simulink model "KF"  (R2021b)
settings: Solver=VariableStepAuto  StartTime=0.0  StopTime=10.0  RelTol=1e-3
values from neighbouring files (symbols this model uses):
  AA = [0 1; g/L 0]    [simConstants.m]
  BB = [0; -1/L]    [simConstants.m]
  CC = [1 0]    [simConstants.m]
  K = W * CC' / V2    [simConstants.m]
libraries: simulink_extras x4
settings Model: Creator=logan  LastModifiedBy=logan

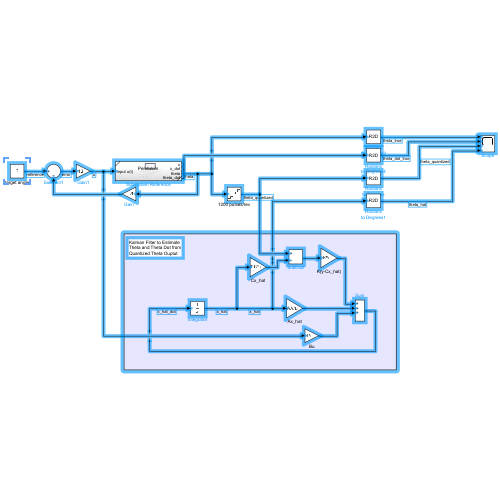
[thumbnail: Simulink's stored preview of the top-level diagram]
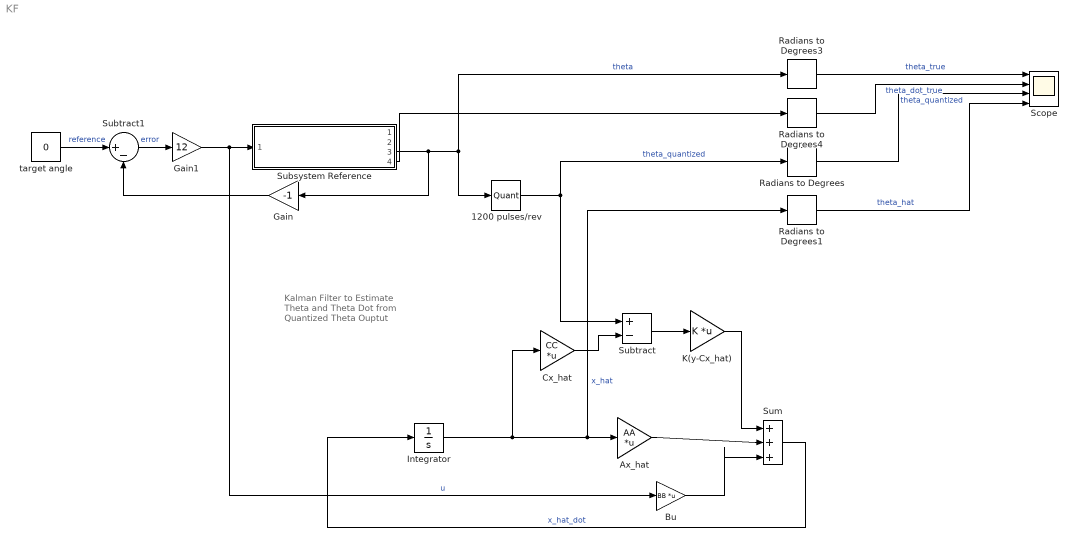
== system KF ==
  note: Kalman Filter to Estimate
      | Theta and Theta Dot from
      | Quantized Theta Ouptut
  1200 pulses/rev : Quantizer  QuantizationInterval=(2*pi)/1200
  Ax_hat : Gain  Gain=AA  Multiplication=Matrix(K*u)
  Bu : Gain  Gain=BB  Multiplication=Matrix(K*u)
  Cx_hat : Gain  Gain=CC  Multiplication=Matrix(K*u)
  Gain : Gain  Gain=-1
  Gain1 : Gain  Gain=12
  Integrator : Integrator
  K(y-Cx_hat) : Gain  Gain=K  Multiplication=Matrix(K*u)
  Radians to Degrees{,1,3..4} (4 alike) : simulink_extras/Transformations/Radians to Degrees
  Scope : Scope  NumInputPorts=4
  Subsystem Reference : Subsystem  ReferencedSubsystem=Pendulum
  Subtract : Sum  Inputs=+-
  Subtract1 : Sum  Inputs=|+-
  Sum : Sum  Inputs=+++|
  target angle : Constant  Value=0  OutDataTypeStr=Inherit: Inherit via back propagation
  wires:
  Subsystem Reference/3 -> Gain/1, Radians to Degrees3/1, 1200 pulses/rev/1  "theta"
  1200 pulses/rev/1 -> Subtract/1, Radians to Degrees/1  "theta_quantized"
  Integrator/1 -> Radians to Degrees1/1, Ax_hat/1, Cx_hat/1  "x_hat"
  Sum/1 -> Integrator/1  "x_hat_dot"
  Subtract/1 -> K(y-Cx_hat)/1
  Cx_hat/1 -> Subtract/2
  K(y-Cx_hat)/1 -> Sum/1
  Ax_hat/1 -> Sum/2
  Gain/1 -> Subtract1/2
  target angle/1 -> Subtract1/1  "reference"
  Gain1/1 -> Bu/1, Subsystem Reference/1  "u"
  Subtract1/1 -> Gain1/1  "error"
  Radians to Degrees/1 -> Scope/3  "theta_quantized"
  Radians to Degrees1/1 -> Scope/4  "theta_hat"
  Radians to Degrees3/1 -> Scope/1  "theta_true"
  Bu/1 -> Sum/3
  Subsystem Reference/4 -> Radians to Degrees4/1
  Radians to Degrees4/1 -> Scope/2  "theta_dot_true"
